simulink model "MotionControl"  (R2024b)
settings: Solver=VariableStepAuto  StartTime=0.0  StopTime=10.0  RelTol=1e-3
model workspace (MAT data in the model file):
  DesLinVel = Simulink.Parameter
  DesLinVel.Value = 0.3
  DesLinVel.Complexity = 'real'
  DesLinVel.Dimensions = [1 1]
  DesLinVel.DataType = 'auto'
  LookaheadDist = Simulink.Parameter
  LookaheadDist.Value = 2
  LookaheadDist.Complexity = 'real'
  LookaheadDist.Dimensions = [1 1]
  LookaheadDist.DataType = 'auto'
values from neighbouring files (symbols this model uses):
  waypoints = 5.0 6.0 7.0 8.0 9.0 10.0 11.0 12.0 13.0 14.0 15.0 16.0 17.0 18.0 19.0 20.0 21.0 22.0 23.0 24.0 25.0 26.0 27.0 28.0 29.0 30.0 31.0 32.0 33.0 34.0 35.0 36.0 37.0 38.0 39.0 40.0 41.0 42.0 43.0 44.0 45.0 46.0 47.0 48.0 49.0 50.0 51.0 52.0 53.0 54.0 55.0 56.0 57.0 58.0 59.0 60.0 61.0 62.0 63.0 64.0 65.0 66.0 67.0 68.0 69.0 70.0 71.0 72.0 73.0 74.0 75.0 76.0 77.0 78.0 79.0 80.0 81.0 82.0 83.0 84.0 85.0    [DataDictionary.sldd]
libraries: robotalgslib x1
settings Model: DataDictionary=DataDictionary.sldd  ParameterArgumentNames=DesLinVel,LookaheadDist  Creator=charber  LastModifiedBy=tsamak

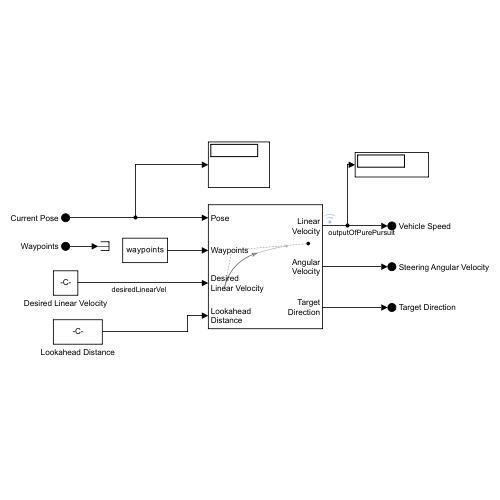
[thumbnail: Simulink's stored preview of the top-level diagram]
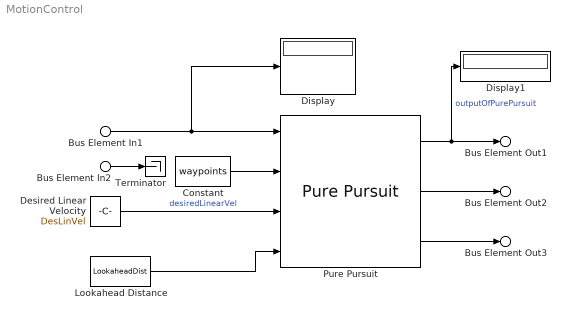
== system MotionControl ==
  Bus Element In1 : Inport  PortName=Current Pose
  Bus Element In2 : Inport  Port=2  PortName=Waypoints
  Constant : Constant  Value=waypoints
  Desired Linear Velocity : Constant  Value=DesLinVel
  Display : Display
  Display1 : Display
  Lookahead Distance : Constant  Value=LookaheadDist
  Pure Pursuit : robotalgslib/Pure Pursuit  DesiredLinearVelocityPort=on  DesiredLinearVelocity=0.3  MaxAngularVelocity=1.0  LookaheadDistancePort=on  LookaheadDistance=2.0  TargetDirPort=on  SimulateUsing=Code generation
  Terminator : Terminator
  Bus Element Out1 : Outport  PortName=Vehicle Speed
  Bus Element Out2 : Outport  Port=2  PortName=Steering Angular Velocity
  Bus Element Out3 : Outport  Port=3  PortName=Target Direction
  wires:
  Lookahead Distance/1 -> Pure Pursuit/4
  Bus Element In2/1 -> Terminator/1
  Pure Pursuit/1 -> Display1/1, Bus Element Out1/1  "outputOfPurePursuit"
  Pure Pursuit/2 -> Bus Element Out2/1
  Pure Pursuit/3 -> Bus Element Out3/1
  Constant/1 -> Pure Pursuit/2
  Desired Linear Velocity/1 -> Pure Pursuit/3  "desiredLinearVel"
  Bus Element In1/1 -> Display/1, Pure Pursuit/1
